simulink model "SimMod"  (R2021a)
settings: Solver=VariableStepAuto  StartTime=0.0  StopTime=20  RelTol=1e-3
model workspace (MAT data in the model file):
  d = [1  1  1  5  5  8; 2  2  3  3  6  6; 1  4  4  4  5  7; 2  2  6  6  7  8; 3  4  5  7  8  8]
  seed = 1234
libraries: simulink x1, rllib x1
settings Model: OrderedModelArguments=off  Creator=mtearle  LastModifiedBy=pawel
settings SolverCC: AlgebraicLoopSolver=TrustRegion
settings DebuggingCC: SFMachineParentedDataDiag=warning

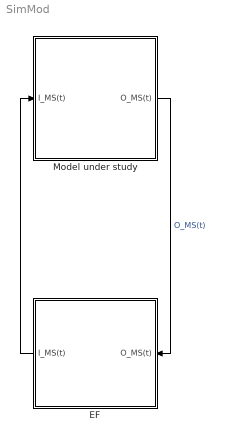
== system SimMod ==
  EF : Subsystem
  Model under study : Subsystem
  wires:
  Model under study/1(O_MS(t)) -> EF/1(O_MS(t))  "O_MS(t)"
  EF/1(I_MS(t)) -> Model under study/1(I_MS(t))

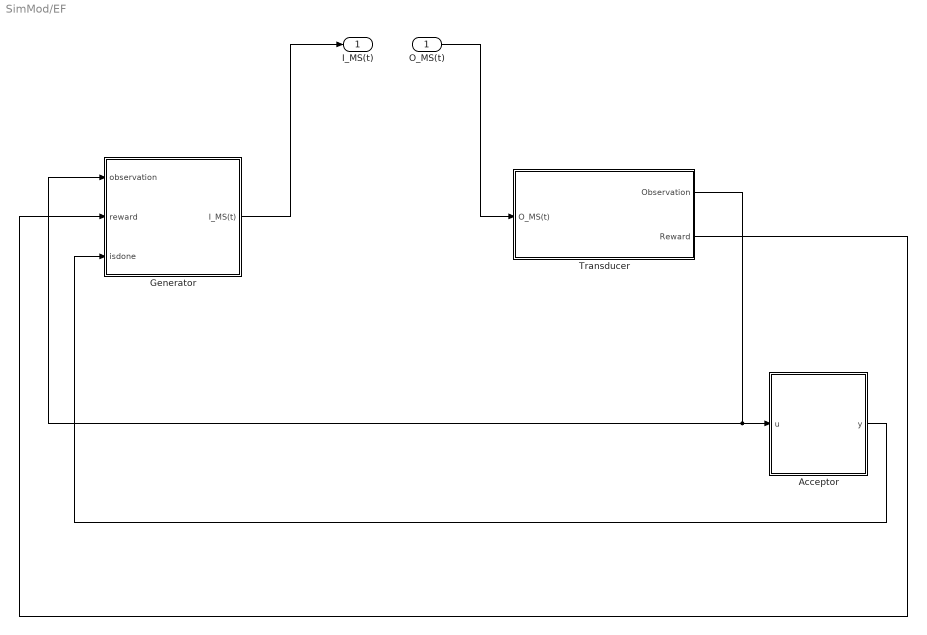
== system SimMod/EF ==
  O_MS(t) : Inport
  Acceptor : Subsystem
  Generator : Subsystem
  Transducer : Subsystem
  I_MS(t) : Outport
  wires:
  Transducer/1(Observation) -> Acceptor/1(u), Generator/1(observation)
  Transducer/2(Reward) -> Generator/2(reward)
  O_MS(t)/1 -> Transducer/1(O_MS(t))
  Acceptor/1(y) -> Generator/3(isdone)
  Generator/1(I_MS(t)) -> I_MS(t)/1

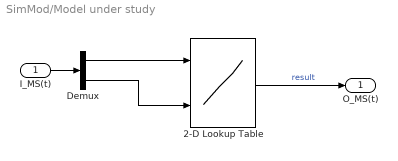
== system SimMod/Model under study ==
  I_MS(t) : Inport
  2-D Lookup Table : Lookup_n-D  BreakpointsSpecification=Even spacing  BreakpointsForDimension1=[1:3]  BreakpointsForDimension2=[1:3]  Table=d  InternalRulePriority=Speed  RndMeth=Simplest  InputSameDT=on
      settings: InputPortMap=u0,u1
  Demux : Demux  Outputs=2
  O_MS(t) : Outport
  wires:
  2-D Lookup Table/1 -> O_MS(t)/1  "result"
  I_MS(t)/1 -> Demux/1
  Demux/1 -> 2-D Lookup Table/1
  Demux/2 -> 2-D Lookup Table/2

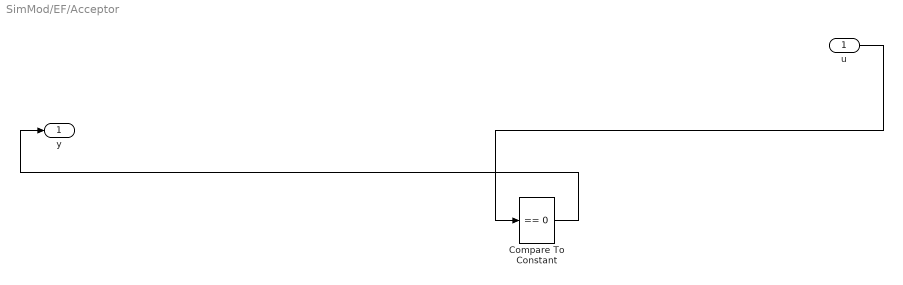
== system SimMod/EF/Acceptor ==
  u : Inport
  Compare To Constant : simulink/Logic and Bit Operations/Compare To Constant  relop===  const=0  OutDataTypeStr=boolean
  y : Outport
  wires:
  u/1 -> Compare To Constant/1
  Compare To Constant/1 -> y/1

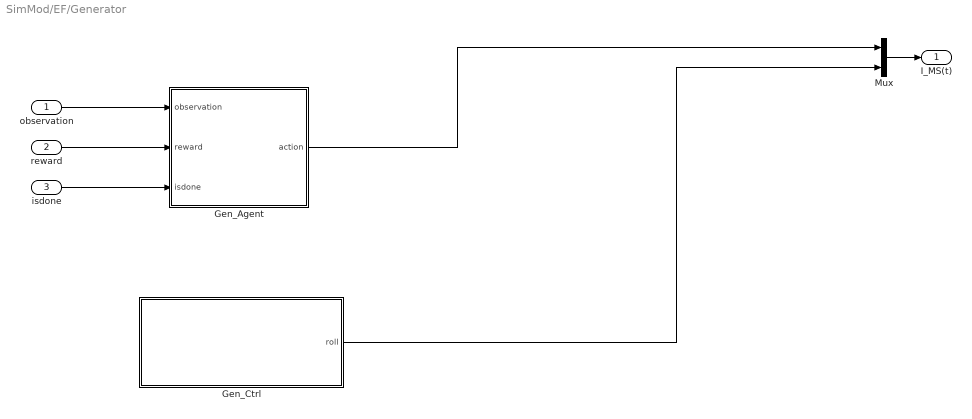
== system SimMod/EF/Generator ==
  observation : Inport
  reward : Inport  Port=2
  isdone : Inport  Port=3
  Gen_Agent : Subsystem
  Gen_Ctrl : Subsystem
  Mux : Mux  Inputs=2
  I_MS(t) : Outport
  wires:
  Mux/1 -> I_MS(t)/1
  observation/1 -> Gen_Agent/1(observation)
  reward/1 -> Gen_Agent/2(reward)
  isdone/1 -> Gen_Agent/3(isdone)
  Gen_Agent/1(action) -> Mux/1
  Gen_Ctrl/1(roll) -> Mux/2

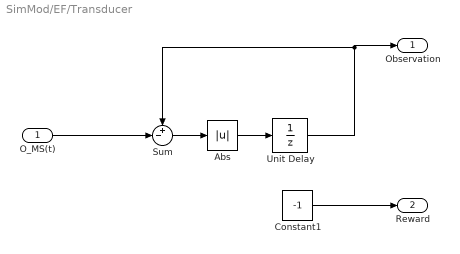
== system SimMod/EF/Transducer ==
  O_MS(t) : Inport
  Abs : Abs
  Constant1 : Constant  Value=-1
  Sum : Sum  Inputs=+-|
  Unit Delay : UnitDelay  InitialCondition=randi(20)  HasFrameUpgradeWarning=on
  Observation : Outport
  Reward : Outport  Port=2
  wires:
  Unit Delay/1 -> Observation/1, Sum/1
  Sum/1 -> Abs/1
  Abs/1 -> Unit Delay/1
  Constant1/1 -> Reward/1
  O_MS(t)/1 -> Sum/2

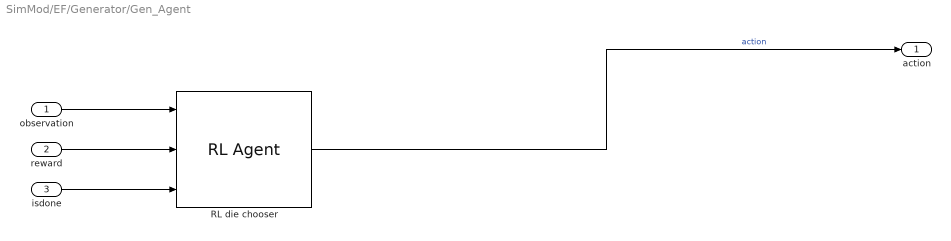
== system SimMod/EF/Generator/Gen_Agent ==
  observation : Inport
  reward : Inport  Port=2
  isdone : Inport  Port=3
  RL die chooser : rllib/RL Agent  Agent=agent  ExternalActionAsInput=off  ProvideCumRwd=off  TreatAsDirectFeedthrough=on
  action : Outport
  wires:
  reward/1 -> RL die chooser/2
  isdone/1 -> RL die chooser/3
  observation/1 -> RL die chooser/1
  RL die chooser/1 -> action/1  "action"

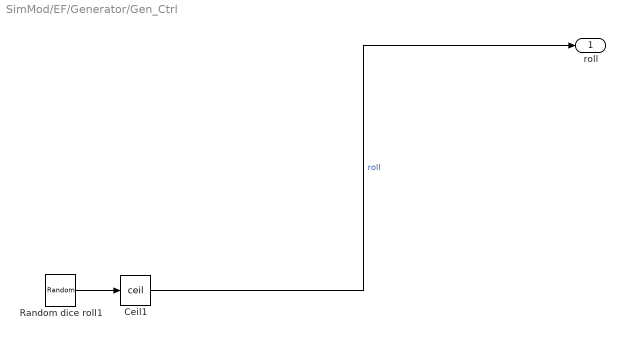
== system SimMod/EF/Generator/Gen_Ctrl ==
  Ceil1 : Rounding  Operator=ceil
  Random dice roll1 : UniformRandomNumber  Minimum=0  Maximum=size(d,2)  Seed=seed  SampleTime=1
  roll : Outport
  wires:
  Random dice roll1/1 -> Ceil1/1
  Ceil1/1 -> roll/1  "roll"
